simulink model "Standard_Test_Signal"  (R2021a)
settings: Solver=VariableStepAuto  StartTime=0.0  StopTime=10.0  RelTol=1e-3
libraries: simulink x1
settings Model: Creator=lenovo  LastModifiedBy=lenovo

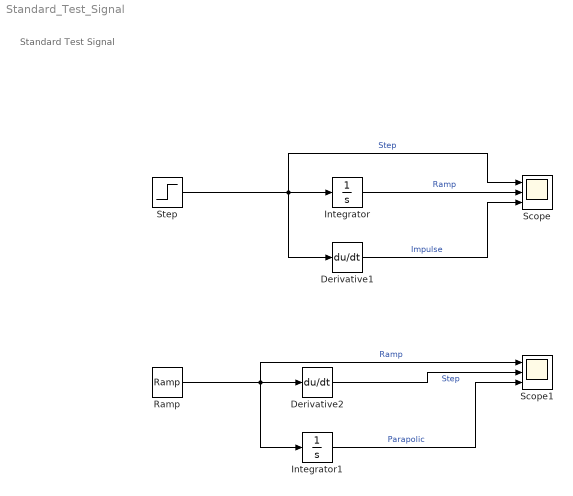
== system Standard_Test_Signal ==
  note: Standard Test Signal
  Derivative1 : Derivative
  Derivative2 : Derivative
  Integrator : Integrator
  Integrator1 : Integrator
  Ramp : simulink/Sources/Ramp  slope=1  start=0  InitialOutput=0
  Scope : Scope  NumInputPorts=3
  Scope1 : Scope  NumInputPorts=3
  Step : Step  SampleTime=0
  wires:
  Step/1 -> Derivative1/1, Integrator/1, Scope/1  "Step"
  Integrator/1 -> Scope/2  "Ramp"
  Derivative1/1 -> Scope/3  "Impulse"
  Ramp/1 -> Integrator1/1, Scope1/1, Derivative2/1  "Ramp"
  Derivative2/1 -> Scope1/2  "Step"
  Integrator1/1 -> Scope1/3  "Parapolic"
